simulink model "Unity_6DOFMICO_Inversekine_v8"  (R2019b)
settings: Solver=ode5  StartTime=0.0  StopTime=inf  FixedStep=0.001  RelTol=1e-3
undefined symbols (not defined in the file): f, Sub02MIHM
libraries: instrumentlib x10, simulink x10, dspnetwork x6, powerlib_meascontrol x3, dspsrcs4 x1
(part 3 of 3)

== matlab function Unity_6DOFMICO_Inversekine_v8/Trajectory Planning/Iterator/Subsystem/MATLAB Function4 ==
  data: val input; out output; x input; y input; z input
function out  = fcn(val,x,y,z)

if val ==1 & x<0.5 & x>=-0.5
    out=1;
elseif val==2 & x<0.35 & x>-0.35
    out=2;
elseif val==3 & y<0.35 & y>=-0.17
    out=3;
elseif val==4 & y<=0.25 & y>-0.25
    out=4;
elseif val==5 & z<0.25 & z>=-0.25
    out=5;
elseif val==6 & z<=0.35 & z>-0.35
    out=6;
elseif val==7
    out=7;
else val==8
    out=8;

end
end
